simulink model "Energy"  (Simulink 7.7)
settings: Solver=ode45  StartTime=0.0  StopTime=274.7493  RelTol=1e-3
settings Model: Creator=baqumau  LastModifiedBy=baqumau

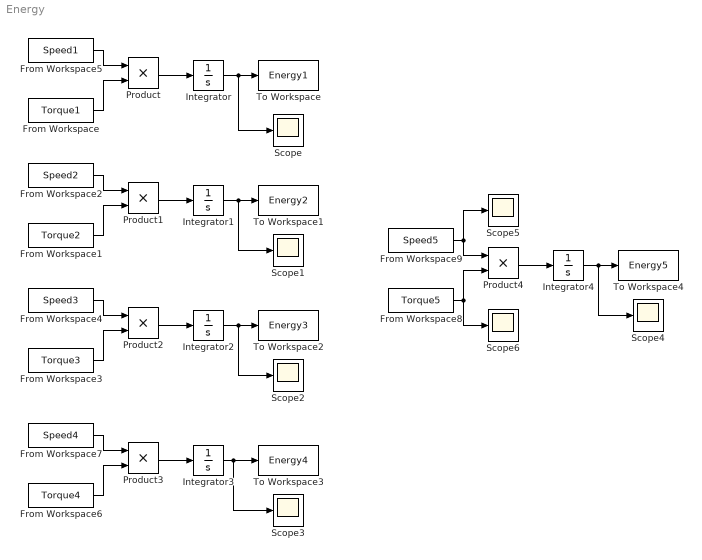
== system Energy ==
  From Workspace : FromWorkspace  VariableName=Torque1  SampleTime=0
  From Workspace1 : FromWorkspace  VariableName=Torque2  SampleTime=0
  From Workspace2 : FromWorkspace  VariableName=Speed2  SampleTime=0
  From Workspace3 : FromWorkspace  VariableName=Torque3  SampleTime=0
  From Workspace4 : FromWorkspace  VariableName=Speed3  SampleTime=0
  From Workspace5 : FromWorkspace  VariableName=Speed1  SampleTime=0
  From Workspace6 : FromWorkspace  VariableName=Torque4  SampleTime=0
  From Workspace7 : FromWorkspace  VariableName=Speed4  SampleTime=0
  From Workspace8 : FromWorkspace  VariableName=Torque5  SampleTime=0
  From Workspace9 : FromWorkspace  VariableName=Speed5  SampleTime=0
  Integrator{,1..4} (5 alike) : Integrator
  Product{,1..4} (5 alike) : Product  RndMeth=Zero
  Scope{,1..6} (7 alike) : Scope
      Scope2 settings: SaveName=ScopeData2
      Scope3 settings: SaveName=ScopeData3
      Scope4 settings: SaveName=ScopeData4
      Scope5 settings: SaveName=ScopeData5
      Scope6 settings: SaveName=ScopeData6
  To Workspace : ToWorkspace  VariableName=Energy1  SampleTime=-1  SaveFormat=Structure With Time
  To Workspace1 : ToWorkspace  VariableName=Energy2  SampleTime=-1  SaveFormat=Structure With Time
  To Workspace2 : ToWorkspace  VariableName=Energy3  SampleTime=-1  SaveFormat=Structure With Time
  To Workspace3 : ToWorkspace  VariableName=Energy4  SampleTime=-1  SaveFormat=Structure With Time
  To Workspace4 : ToWorkspace  VariableName=Energy5  SampleTime=-1  SaveFormat=Structure With Time
  wires:
  From Workspace5/1 -> Product/1
  From Workspace/1 -> Product/2
  Product/1 -> Integrator/1
  Integrator/1 -> To Workspace/1, Scope/1
  From Workspace2/1 -> Product1/1
  From Workspace1/1 -> Product1/2
  Product1/1 -> Integrator1/1
  Integrator1/1 -> To Workspace1/1, Scope1/1
  From Workspace4/1 -> Product2/1
  From Workspace3/1 -> Product2/2
  Product2/1 -> Integrator2/1
  Integrator2/1 -> To Workspace2/1, Scope2/1
  From Workspace7/1 -> Product3/1
  From Workspace6/1 -> Product3/2
  Product3/1 -> Integrator3/1
  Integrator3/1 -> To Workspace3/1, Scope3/1
  From Workspace9/1 -> Product4/1, Scope5/1
  From Workspace8/1 -> Product4/2, Scope6/1
  Product4/1 -> Integrator4/1
  Integrator4/1 -> To Workspace4/1, Scope4/1
